simulink model "NLGuidance_12B_with_contracts_SLDV_tmp"  (Simulink 9.0)
settings: Solver=ode3  StartTime=0.0  StopTime=10.0  FixedStep=.02  RelTol=1e-3  EnableMultiTasking=on
model workspace (MAT data in the model file):
  ContractValidatorBlocksMap = containers.Map
  ContractValidatorBlocksMap.serialization.keys = {'NLGuidance_12B/contract/validator', 'NLGuidance_12B_with_contracts/contract/validator'}
  ContractValidatorBlocksMap.serialization.values{1}.block = 'NLGuidance_12B/contract/validator'
  ContractValidatorBlocksMap.serialization.values{1}.assumePorts = 2
  ContractValidatorBlocksMap.serialization.values{1}.guaranteePorts = 6
  ContractValidatorBlocksMap.serialization.values{1}.modeBlocksPorts = 0
  ContractValidatorBlocksMap.serialization.values{1}.portHandles.Inport = [1044.00036621 1045.00036621 1046.00036621 1047.00036621 1048.00036621 1049.00036621 1050.00036621 1051.00036621]
  ContractValidatorBlocksMap.serialization.values{1}.portHandles.Outport = 1052.00036621
  ContractValidatorBlocksMap.serialization.values{1}.portHandles.Enable = []
  ContractValidatorBlocksMap.serialization.values{1}.portHandles.Trigger = []
  ContractValidatorBlocksMap.serialization.values{1}.portHandles.State = []
  ContractValidatorBlocksMap.serialization.values{1}.portHandles.LConn = []
  ContractValidatorBlocksMap.serialization.values{1}.portHandles.RConn = []
  ContractValidatorBlocksMap.serialization.values{1}.portHandles.Ifaction = []
  ContractValidatorBlocksMap.serialization.values{1}.portHandles.Reset = []
  ContractValidatorBlocksMap.serialization.values{1}.portConnectivity(1).Type = '1'
  ContractValidatorBlocksMap.serialization.values{1}.portConnectivity(1).Position = [365 -130]
  ContractValidatorBlocksMap.serialization.values{1}.portConnectivity(1).SrcBlock = 945.000488281
  ContractValidatorBlocksMap.serialization.values{1}.portConnectivity(1).SrcPort = 0
  ContractValidatorBlocksMap.serialization.values{1}.portConnectivity(1).DstBlock = []
  ContractValidatorBlocksMap.serialization.values{1}.portConnectivity(1).DstPort = []
  ContractValidatorBlocksMap.serialization.values{1}.portConnectivity(2).Type = '2'
  ContractValidatorBlocksMap.serialization.values{1}.portConnectivity(2).Position = [365 -40]
  ContractValidatorBlocksMap.serialization.values{1}.portConnectivity(2).SrcBlock = 953.000488281
  ContractValidatorBlocksMap.serialization.values{1}.portConnectivity(2).SrcPort = 0
  ContractValidatorBlocksMap.serialization.values{1}.portConnectivity(2).DstBlock = []
  ContractValidatorBlocksMap.serialization.values{1}.portConnectivity(2).DstPort = []
  ContractValidatorBlocksMap.serialization.values{1}.portConnectivity(3).Type = '3'
  ContractValidatorBlocksMap.serialization.values{1}.portConnectivity(3).Position = [365 50]
  ContractValidatorBlocksMap.serialization.values{1}.portConnectivity(3).SrcBlock = 932.000488281
  ContractValidatorBlocksMap.serialization.values{1}.portConnectivity(3).SrcPort = 0
  ContractValidatorBlocksMap.serialization.values{1}.portConnectivity(3).DstBlock = []
  ContractValidatorBlocksMap.serialization.values{1}.portConnectivity(3).DstPort = []
  ContractValidatorBlocksMap.serialization.values{1}.portConnectivity(4).Type = '4'
  ContractValidatorBlocksMap.serialization.values{1}.portConnectivity(4).Position = [365 140]
  ContractValidatorBlocksMap.serialization.values{1}.portConnectivity(4).SrcBlock = 766.000488281
  ContractValidatorBlocksMap.serialization.values{1}.portConnectivity(4).SrcPort = 0
  ContractValidatorBlocksMap.serialization.values{1}.portConnectivity(4).DstBlock = []
  ContractValidatorBlocksMap.serialization.values{1}.portConnectivity(4).DstPort = []
  ContractValidatorBlocksMap.serialization.values{1}.portConnectivity(5).Type = '5'
  ContractValidatorBlocksMap.serialization.values{1}.portConnectivity(5).Position = [365 230]
  ContractValidatorBlocksMap.serialization.values{1}.portConnectivity(5).SrcBlock = 803.000732422
  ContractValidatorBlocksMap.serialization.values{1}.portConnectivity(5).SrcPort = 0
  ContractValidatorBlocksMap.serialization.values{1}.portConnectivity(5).DstBlock = []
  ContractValidatorBlocksMap.serialization.values{1}.portConnectivity(5).DstPort = []
  ContractValidatorBlocksMap.serialization.values{1}.portConnectivity(6).Type = '6'
  ContractValidatorBlocksMap.serialization.values{1}.portConnectivity(6).Position = [365 320]
  ContractValidatorBlocksMap.serialization.values{1}.portConnectivity(6).SrcBlock = 813.000732422
  ContractValidatorBlocksMap.serialization.values{1}.portConnectivity(6).SrcPort = 0
  ContractValidatorBlocksMap.serialization.values{1}.portConnectivity(6).DstBlock = []
  ContractValidatorBlocksMap.serialization.values{1}.portConnectivity(6).DstPort = []
  ContractValidatorBlocksMap.serialization.values{1}.portConnectivity(7).Type = '7'
  ContractValidatorBlocksMap.serialization.values{1}.portConnectivity(7).Position = [365 410]
  ContractValidatorBlocksMap.serialization.values{1}.portConnectivity(7).SrcBlock = 874.000732422
  ContractValidatorBlocksMap.serialization.values{1}.portConnectivity(7).SrcPort = 0
  ContractValidatorBlocksMap.serialization.values{1}.portConnectivity(7).DstBlock = []
  ContractValidatorBlocksMap.serialization.values{1}.portConnectivity(7).DstPort = []
  ContractValidatorBlocksMap.serialization.values{1}.portConnectivity(8).Type = '8'
  ContractValidatorBlocksMap.serialization.values{1}.portConnectivity(8).Position = [365 500]
  ContractValidatorBlocksMap.serialization.values{1}.portConnectivity(8).SrcBlock = 920.000732422
  ContractValidatorBlocksMap.serialization.values{1}.portConnectivity(8).SrcPort = 0
  ContractValidatorBlocksMap.serialization.values{1}.portConnectivity(8).DstBlock = []
  ContractValidatorBlocksMap.serialization.values{1}.portConnectivity(8).DstPort = []
  ContractValidatorBlocksMap.serialization.values{1}.portConnectivity(9).Type = '1'
  ContractValidatorBlocksMap.serialization.values{1}.portConnectivity(9).Position = [510 185]
  ContractValidatorBlocksMap.serialization.values{1}.portConnectivity(9).SrcBlock = []
  ContractValidatorBlocksMap.serialization.values{1}.portConnectivity(9).SrcPort = []
  ContractValidatorBlocksMap.serialization.values{1}.portConnectivity(9).DstBlock = 962.000488281
  ContractValidatorBlocksMap.serialization.values{1}.portConnectivity(9).DstPort = 0
  ContractValidatorBlocksMap.serialization.values{2}.block = 'NLGuidance_12B_with_contracts/contract/validator'
  ContractValidatorBlocksMap.serialization.values{2}.assumePorts = 2
  ContractValidatorBlocksMap.serialization.values{2}.guaranteePorts = 6
  ContractValidatorBlocksMap.serialization.values{2}.modeBlocksPorts = 0
  ContractValidatorBlocksMap.serialization.values{2}.portHandles.Inport = [4812.00012207 4813.00012207 4814.00012207 4815.00012207 4816.00012207 4817.00012207 4818.00012207 4819.00012207]
  ContractValidatorBlocksMap.serialization.values{2}.portHandles.Outport = 4820.00012207
  ContractValidatorBlocksMap.serialization.values{2}.portHandles.Enable = []
  ContractValidatorBlocksMap.serialization.values{2}.portHandles.Trigger = []
  ContractValidatorBlocksMap.serialization.values{2}.portHandles.State = []
  ContractValidatorBlocksMap.serialization.values{2}.portHandles.LConn = []
  ContractValidatorBlocksMap.serialization.values{2}.portHandles.RConn = []
  ContractValidatorBlocksMap.serialization.values{2}.portHandles.Ifaction = []
  ContractValidatorBlocksMap.serialization.values{2}.portHandles.Reset = []
  ContractValidatorBlocksMap.serialization.values{2}.portConnectivity(1).Type = '1'
  ContractValidatorBlocksMap.serialization.values{2}.portConnectivity(1).Position = [365 -130]
  ContractValidatorBlocksMap.serialization.values{2}.portConnectivity(1).SrcBlock = 4713.00012207
  ContractValidatorBlocksMap.serialization.values{2}.portConnectivity(1).SrcPort = 0
  ContractValidatorBlocksMap.serialization.values{2}.portConnectivity(1).DstBlock = []
  ContractValidatorBlocksMap.serialization.values{2}.portConnectivity(1).DstPort = []
  ContractValidatorBlocksMap.serialization.values{2}.portConnectivity(2).Type = '2'
  ContractValidatorBlocksMap.serialization.values{2}.portConnectivity(2).Position = [365 -40]
  ContractValidatorBlocksMap.serialization.values{2}.portConnectivity(2).SrcBlock = 4721.00012207
  ContractValidatorBlocksMap.serialization.values{2}.portConnectivity(2).SrcPort = 0
  ContractValidatorBlocksMap.serialization.values{2}.portConnectivity(2).DstBlock = []
  ContractValidatorBlocksMap.serialization.values{2}.portConnectivity(2).DstPort = []
  ContractValidatorBlocksMap.serialization.values{2}.portConnectivity(3).Type = '3'
  ContractValidatorBlocksMap.serialization.values{2}.portConnectivity(3).Position = [365 50]
  ContractValidatorBlocksMap.serialization.values{2}.portConnectivity(3).SrcBlock = 4700.00012207
  ContractValidatorBlocksMap.serialization.values{2}.portConnectivity(3).SrcPort = 0
  ContractValidatorBlocksMap.serialization.values{2}.portConnectivity(3).DstBlock = []
  ContractValidatorBlocksMap.serialization.values{2}.portConnectivity(3).DstPort = []
  ContractValidatorBlocksMap.serialization.values{2}.portConnectivity(4).Type = '4'
  ContractValidatorBlocksMap.serialization.values{2}.portConnectivity(4).Position = [365 140]
  ContractValidatorBlocksMap.serialization.values{2}.portConnectivity(4).SrcBlock = 4534.00012207
  ContractValidatorBlocksMap.serialization.values{2}.portConnectivity(4).SrcPort = 0
  ContractValidatorBlocksMap.serialization.values{2}.portConnectivity(4).DstBlock = []
  ContractValidatorBlocksMap.serialization.values{2}.portConnectivity(4).DstPort = []
  ContractValidatorBlocksMap.serialization.values{2}.portConnectivity(5).Type = '5'
  ContractValidatorBlocksMap.serialization.values{2}.portConnectivity(5).Position = [365 230]
  ContractValidatorBlocksMap.serialization.values{2}.portConnectivity(5).SrcBlock = 4571.00012207
  ContractValidatorBlocksMap.serialization.values{2}.portConnectivity(5).SrcPort = 0
  ContractValidatorBlocksMap.serialization.values{2}.portConnectivity(5).DstBlock = []
  ContractValidatorBlocksMap.serialization.values{2}.portConnectivity(5).DstPort = []
  ContractValidatorBlocksMap.serialization.values{2}.portConnectivity(6).Type = '6'
  ContractValidatorBlocksMap.serialization.values{2}.portConnectivity(6).Position = [365 320]
  ContractValidatorBlocksMap.serialization.values{2}.portConnectivity(6).SrcBlock = 4581.00012207
  ContractValidatorBlocksMap.serialization.values{2}.portConnectivity(6).SrcPort = 0
  ContractValidatorBlocksMap.serialization.values{2}.portConnectivity(6).DstBlock = []
  ContractValidatorBlocksMap.serialization.values{2}.portConnectivity(6).DstPort = []
  ContractValidatorBlocksMap.serialization.values{2}.portConnectivity(7).Type = '7'
  ContractValidatorBlocksMap.serialization.values{2}.portConnectivity(7).Position = [365 410]
  ContractValidatorBlocksMap.serialization.values{2}.portConnectivity(7).SrcBlock = 4642.00012207
  ContractValidatorBlocksMap.serialization.values{2}.portConnectivity(7).SrcPort = 0
  ContractValidatorBlocksMap.serialization.values{2}.portConnectivity(7).DstBlock = []
  ContractValidatorBlocksMap.serialization.values{2}.portConnectivity(7).DstPort = []
  ContractValidatorBlocksMap.serialization.values{2}.portConnectivity(8).Type = '8'
  ContractValidatorBlocksMap.serialization.values{2}.portConnectivity(8).Position = [365 500]
  ContractValidatorBlocksMap.serialization.values{2}.portConnectivity(8).SrcBlock = 4688.00012207
  ContractValidatorBlocksMap.serialization.values{2}.portConnectivity(8).SrcPort = 0
  ContractValidatorBlocksMap.serialization.values{2}.portConnectivity(8).DstBlock = []
  ContractValidatorBlocksMap.serialization.values{2}.portConnectivity(8).DstPort = []
  ContractValidatorBlocksMap.serialization.values{2}.portConnectivity(9).Type = '1'
  ContractValidatorBlocksMap.serialization.values{2}.portConnectivity(9).Position = [510 185]
  ContractValidatorBlocksMap.serialization.values{2}.portConnectivity(9).SrcBlock = []
  ContractValidatorBlocksMap.serialization.values{2}.portConnectivity(9).SrcPort = []
  ContractValidatorBlocksMap.serialization.values{2}.portConnectivity(9).DstBlock = 4730.00012207
  ContractValidatorBlocksMap.serialization.values{2}.portConnectivity(9).DstPort = 0
  ContractValidatorBlocksMap.serialization.uniformity = 0
  ContractValidatorBlocksMap.serialization.keyType = 'char'
  ContractValidatorBlocksMap.serialization.valueType = 'any'
libraries: sldvlib x9, simulink x6
settings Model: Creator=elliocm  LastModifiedBy=hbourbou
settings DataIOCC: LimitDataPoints=on  SignalLoggingSaveFormat=ModelDataLogs
settings OptimizationCC: ExpressionDepthLimit=2147483647
settings DebuggingCC: SolverPrmCheckMsg=warning  MultiTaskDSMMsg=warning  MultiTaskCondExecSysMsg=none  StateNameClashWarn=warning
settings GRTTargetCC: GeneratePreprocessorConditionals=Disable all
settings ConfigComp: DVMode=PropertyProving  DVMaxProcessTime=7200  DVTestSuiteOptimization=CombinedObjectives (Nonlinear Extended)

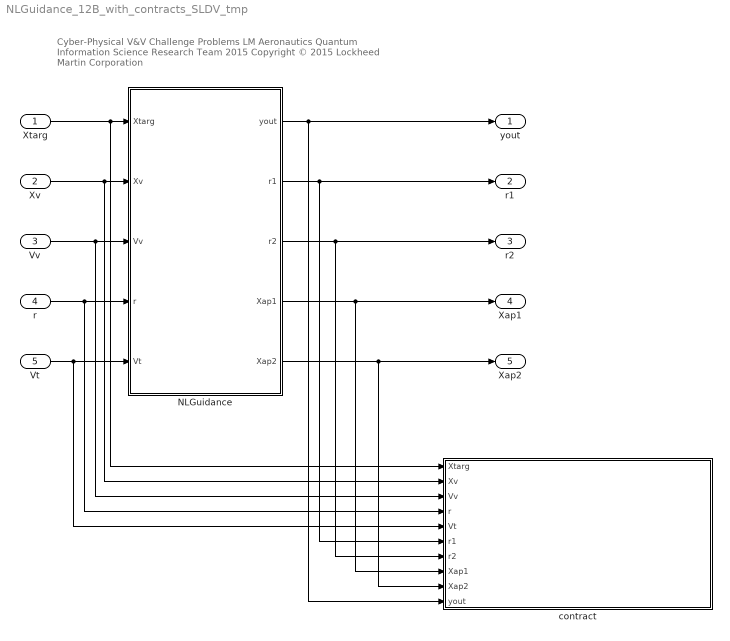
== system NLGuidance_12B_with_contracts_SLDV_tmp ==
  note: Cyber-Physical V&V Challenge Problems
      | LM Aeronautics Quantum Information Science Research Team 2015
      | Copyright © 2015 Lockheed Martin Corporation
  Xtarg : Inport  OutDataTypeStr=double  PortDimensions=3
  Xv : Inport  Port=2  OutDataTypeStr=double  PortDimensions=3
  Vv : Inport  Port=3  OutDataTypeStr=double  PortDimensions=3
  r : Inport  Port=4  OutDataTypeStr=double
  Vt : Inport  Port=5  OutDataTypeStr=double  PortDimensions=3
  NLGuidance : Subsystem
  contract : Subsystem  TreatAsAtomicUnit=on  mask(VerificationSubsystem){}
      settings: CopyFcn=set_param(gcb, 'LinkStatus', 'none');
      mask Display: image(imread('sldvicon_versubsys.png','BackGroundColor',[1 1 1]),'center');
  yout : Outport  VectorParamsAs1DForOutWhenUnconnected=off
  r1 : Outport  Port=2  VectorParamsAs1DForOutWhenUnconnected=off
  r2 : Outport  Port=3  VectorParamsAs1DForOutWhenUnconnected=off
  Xap1 : Outport  Port=4  VectorParamsAs1DForOutWhenUnconnected=off
  Xap2 : Outport  Port=5  VectorParamsAs1DForOutWhenUnconnected=off
  wires:
  NLGuidance/1(yout) -> contract/10(yout), yout/1
  Xv/1 -> contract/2(Xv), NLGuidance/2(Xv)
  Vv/1 -> contract/3(Vv), NLGuidance/3(Vv)
  r/1 -> contract/4(r), NLGuidance/4(r)
  Vt/1 -> contract/5(Vt), NLGuidance/5(Vt)
  Xtarg/1 -> contract/1(Xtarg), NLGuidance/1(Xtarg)
  NLGuidance/3(r2) -> contract/7(r2), r2/1
  NLGuidance/4(Xap1) -> contract/8(Xap1), Xap1/1
  NLGuidance/5(Xap2) -> contract/9(Xap2), Xap2/1
  NLGuidance/2(r1) -> contract/6(r1), r1/1

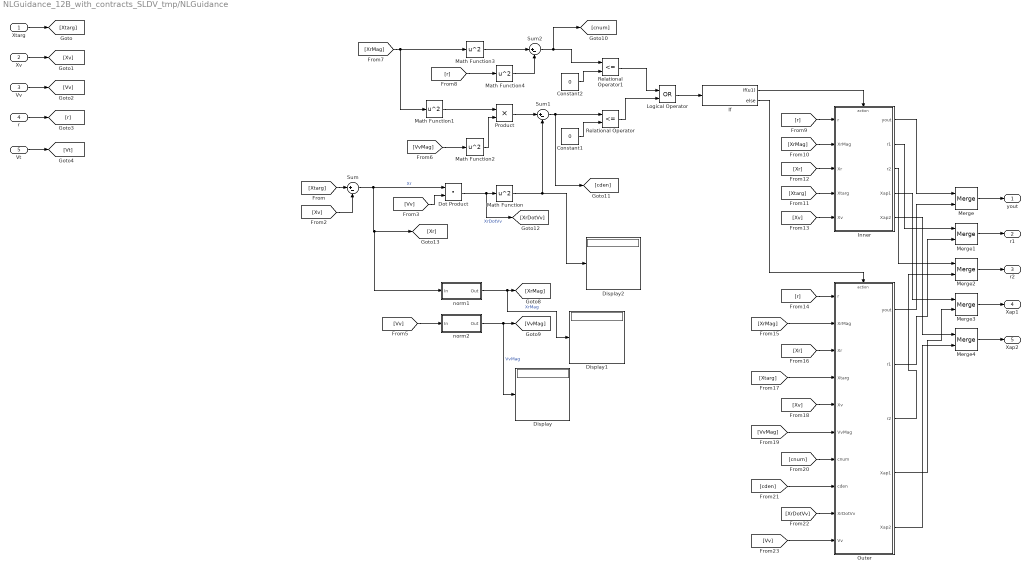
== system NLGuidance_12B_with_contracts_SLDV_tmp/NLGuidance ==
  Xtarg : Inport
  Xv : Inport  Port=2
  Vv : Inport  Port=3
  r : Inport  Port=4
  Vt : Inport  Port=5
  Constant1 : Constant  Value=0
  Constant2 : Constant  Value=0
  Display : Display
  Display1 : Display
  Display2 : Display
  Dot Product : DotProduct  InputSameDT=on  OutDataTypeStr=Inherit: Inherit via internal rule
  If : If  IfExpression=u1
  Inner : Subsystem
  Logical Operator : Logic  Operator=OR  AllPortsSameDT=off  OutDataTypeStr=boolean
  Math Function{,1..4} (5 alike) : Math  Operator=square  SaturateOnIntegerOverflow=on
  Merge{,1..4} (5 alike) : Merge
  Outer : Subsystem
  Product : Product  RndMeth=Zero
  Relational Operator : RelationalOperator  Operator=<=  OutDataTypeStr=boolean  RndMeth=Nearest
  Relational Operator1 : RelationalOperator  Operator=<=  OutDataTypeStr=boolean  RndMeth=Nearest
  Sum : Sum  Inputs=|+-
  Sum1 : Sum  Inputs=|+-
  Sum2 : Sum  Inputs=|+-
  norm1 : Subsystem
  norm2 : Subsystem
  yout : Outport  VectorParamsAs1DForOutWhenUnconnected=off
  r1 : Outport  Port=2  VectorParamsAs1DForOutWhenUnconnected=off
  r2 : Outport  Port=3  VectorParamsAs1DForOutWhenUnconnected=off
  Xap1 : Outport  Port=4  VectorParamsAs1DForOutWhenUnconnected=off
  Xap2 : Outport  Port=5  VectorParamsAs1DForOutWhenUnconnected=off
  wires:
  Xtarg/1 -> [Xtarg]
  Xv/1 -> [Xv]
  Vv/1 -> [Vv]
  r/1 -> [r]
  Vt/1 -> [Vt]
  [Xtarg] -> Sum/1
  [Xv] -> Sum/2
  Sum/1 -> norm1/1(In), [Xr], Dot Product/1  "Xr"
  [Vv] -> Dot Product/2
  Dot Product/1 -> [XrDotVv], Math Function/1  "XrDotVv"
  norm1/1(Out) -> Display1/1, [XrMag]  "XrMag"
  [Vv] -> norm2/1(In)
  norm2/1(Out) -> Display/1, [VvMag]  "VvMag"
  Math Function/1 -> Display2/1, Sum1/2
  [VvMag] -> Math Function2/1
  Math Function1/1 -> Product/1
  Math Function2/1 -> Product/2
  Product/1 -> Sum1/1
  Sum1/1 -> [cden], Relational Operator/1
  Constant1/1 -> Relational Operator/2
  Relational Operator/1 -> Logical Operator/2
  Sum2/1 -> [cnum], Relational Operator1/1
  Constant2/1 -> Relational Operator1/2
  Relational Operator1/1 -> Logical Operator/1
  Math Function3/1 -> Sum2/1
  [XrMag] -> Math Function1/1, Math Function3/1
  Math Function4/1 -> Sum2/2
  [r] -> Math Function4/1
  [r] -> Inner/1(r)
  [XrMag] -> Inner/2(XrMag)
  Logical Operator/1 -> If/1
  [Xtarg] -> Inner/4(Xtarg)
  [Xr] -> Inner/3(Xr)
  [Xv] -> Inner/5(Xv)
  Inner/1(yout) -> Merge/1
  Outer/1(yout) -> Merge/2
  If/1 -> Inner/Action
  If/2 -> Outer/Action
  [r] -> Outer/1(r)
  [XrMag] -> Outer/2(XrMag)
  [Xr] -> Outer/3(Xr)
  [Xtarg] -> Outer/4(Xtarg)
  [Xv] -> Outer/5(Xv)
  [VvMag] -> Outer/6(VvMag)
  [cnum] -> Outer/7(cnum)
  [cden] -> Outer/8(cden)
  [XrDotVv] -> Outer/9(XrDotVv)
  [Vv] -> Outer/10(Vv)
  Merge/1 -> yout/1
  Merge1/1 -> r1/1
  Inner/2(r1) -> Merge1/1
  Outer/2(r1) -> Merge1/2
  Merge2/1 -> r2/1
  Outer/3(r2) -> Merge2/2
  Inner/3(r2) -> Merge2/1
  Merge3/1 -> Xap1/1
  Merge4/1 -> Xap2/1
  Inner/4(Xap1) -> Merge3/1
  Outer/4(Xap1) -> Merge3/2
  Inner/5(Xap2) -> Merge4/1
  Outer/5(Xap2) -> Merge4/2

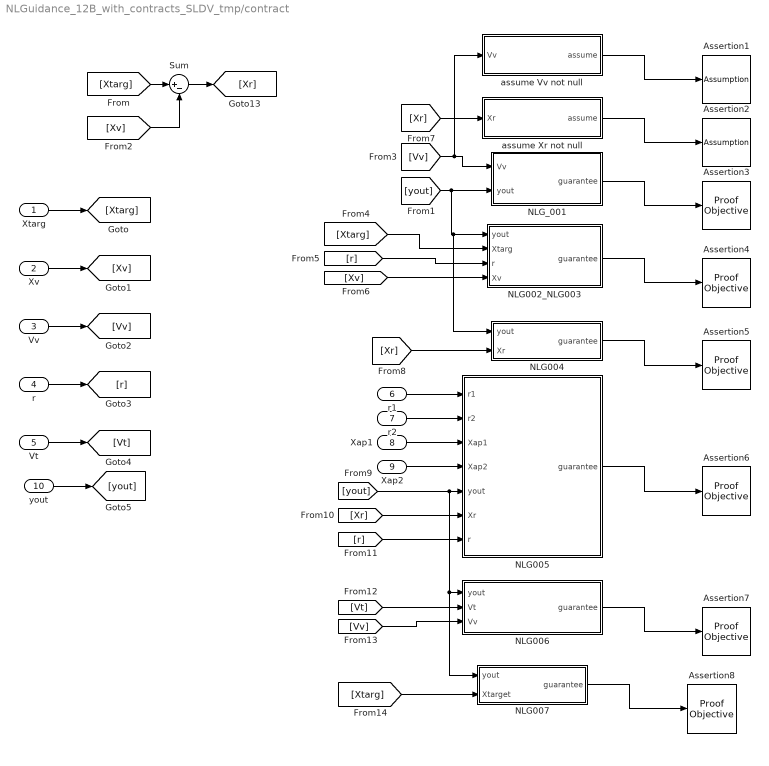
== system NLGuidance_12B_with_contracts_SLDV_tmp/contract ==
  Xtarg : Inport  OutDataTypeStr=double  PortDimensions=3
  Xv : Inport  Port=2  OutDataTypeStr=double  PortDimensions=3
  Vv : Inport  Port=3  OutDataTypeStr=double  PortDimensions=3
  r : Inport  Port=4  OutDataTypeStr=double
  Vt : Inport  Port=5  OutDataTypeStr=double  PortDimensions=3
  r1 : Inport  Port=6
  r2 : Inport  Port=7
  Xap1 : Inport  Port=8
  Xap2 : Inport  Port=9
  yout : Inport  Port=10
  Assertion1 : sldvlib/Objectives and Constraints/Assumption  enabled=on  customAVTBlockType=Assumption  intervals=true  initial=off  dispValues=on  outEnabled=off
      settings: AttributesFormatString=%<intervals>  SourceProductName=Simulink  SourceProductBaseCode=SL
  Assertion2 : sldvlib/Objectives and Constraints/Assumption  enabled=on  customAVTBlockType=Assumption  intervals=true  initial=off  dispValues=on  outEnabled=off
      settings: AttributesFormatString=%<intervals>  SourceProductName=Simulink  SourceProductBaseCode=SL
  Assertion{3..8} (6 alike) : sldvlib/Objectives and Constraints/Proof Objective  enabled=on  customAVTBlockType=Proof Objective  intervals=true  dispValues=on  outEnabled=off  enableStopSim=off
      settings: AttributesFormatString=%<intervals>  SourceProductName=Simulink  SourceProductBaseCode=SL
  NLG002_NLG003 : Subsystem
  NLG004 : Subsystem
  NLG005 : Subsystem
  NLG006 : Subsystem
  NLG007 : Subsystem
  NLG_001 : Subsystem
  Sum : Sum  Inputs=|+-
  assume Vv not null : Subsystem
  assume Xr not null : Subsystem
  wires:
  Xtarg/1 -> [Xtarg]
  Xv/1 -> [Xv]
  Vv/1 -> [Vv]
  Vt/1 -> [Vt]
  r/1 -> [r]
  [Xv] -> Sum/2
  [Xtarg] -> Sum/1
  Sum/1 -> [Xr]
  [yout] -> NLG004/1(yout), NLG002_NLG003/1(yout), NLG_001/2(yout)
  [Vv] -> assume Vv not null/1(Vv), NLG_001/1(Vv)
  yout/1 -> [yout]
  [Xtarg] -> NLG002_NLG003/2(Xtarg)
  [r] -> NLG002_NLG003/3(r)
  [Xv] -> NLG002_NLG003/4(Xv)
  [Xr] -> assume Xr not null/1(Xr)
  [Xr] -> NLG004/2(Xr)
  r1/1 -> NLG005/1(r1)
  r2/1 -> NLG005/2(r2)
  Xap1/1 -> NLG005/3(Xap1)
  Xap2/1 -> NLG005/4(Xap2)
  [yout] -> NLG007/1(yout), NLG006/1(yout), NLG005/5(yout)
  [Xr] -> NLG005/6(Xr)
  [r] -> NLG005/7(r)
  [Vt] -> NLG006/2(Vt)
  [Vv] -> NLG006/3(Vv)
  [Xtarg] -> NLG007/2(Xtarget)
  assume Vv not null/1(assume) -> Assertion1/1
  assume Xr not null/1(assume) -> Assertion2/1
  NLG_001/1(guarantee) -> Assertion3/1
  NLG002_NLG003/1(guarantee) -> Assertion4/1
  NLG004/1(guarantee) -> Assertion5/1
  NLG005/1(guarantee) -> Assertion6/1
  NLG006/1(guarantee) -> Assertion7/1
  NLG007/1(guarantee) -> Assertion8/1

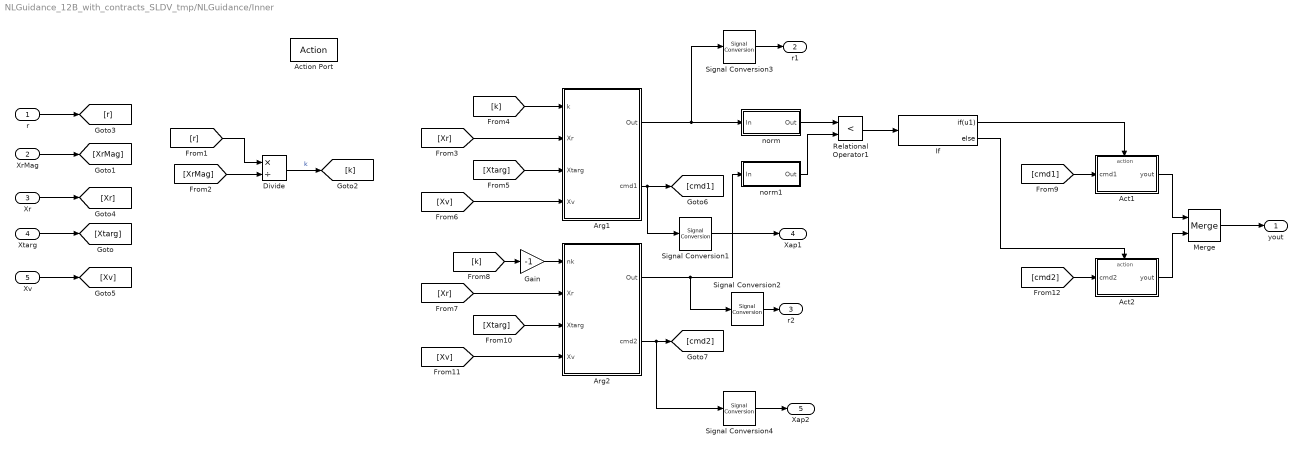
== system NLGuidance_12B_with_contracts_SLDV_tmp/NLGuidance/Inner ==
  r : Inport
  XrMag : Inport  Port=2
  Xr : Inport  Port=3
  Xtarg : Inport  Port=4
  Xv : Inport  Port=5
  Action Port : ActionPort
  Act1 : Subsystem
  Act2 : Subsystem
  Arg1 : Subsystem
  Arg2 : Subsystem
  Divide : Product  Inputs=*/
  Gain : Gain  Gain=-1
  If : If  IfExpression=u1
  Merge : Merge
  Relational Operator1 : RelationalOperator  Operator=<  OutDataTypeStr=boolean  RndMeth=Nearest
  Signal Conversion{1..4} (4 alike) : SignalConversion  OverrideOpt=off
  norm : Subsystem
  norm1 : Subsystem
  yout : Outport  VectorParamsAs1DForOutWhenUnconnected=off
  r1 : Outport  Port=2  VectorParamsAs1DForOutWhenUnconnected=off
  r2 : Outport  Port=3  VectorParamsAs1DForOutWhenUnconnected=off
  Xap1 : Outport  Port=4  VectorParamsAs1DForOutWhenUnconnected=off
  Xap2 : Outport  Port=5  VectorParamsAs1DForOutWhenUnconnected=off
  wires:
  Divide/1 -> [k]  "k"
  r/1 -> [r]
  XrMag/1 -> [XrMag]
  Xtarg/1 -> [Xtarg]
  [r] -> Divide/1
  [XrMag] -> Divide/2
  Xr/1 -> [Xr]
  Xv/1 -> [Xv]
  norm/1(Out) -> Relational Operator1/1
  norm1/1(Out) -> Relational Operator1/2
  Arg1/1(Out) -> Signal Conversion3/1, norm/1(In)
  [k] -> Arg1/1(k)
  [Xr] -> Arg1/2(Xr)
  [Xtarg] -> Arg1/3(Xtarg)
  [Xv] -> Arg1/4(Xv)
  Relational Operator1/1 -> If/1
  [Xr] -> Arg2/2(Xr)
  [Xtarg] -> Arg2/3(Xtarg)
  [Xv] -> Arg2/4(Xv)
  Arg2/1(Out) -> Signal Conversion2/1, norm1/1(In)
  [k] -> Gain/1
  Gain/1 -> Arg2/1(nk)
  Arg1/2(cmd1) -> Signal Conversion1/1, [cmd1]
  [cmd1] -> Act1/1(cmd1)
  [cmd2] -> Act2/1(cmd2)
  Act1/1(yout) -> Merge/1
  Act2/1(yout) -> Merge/2
  Merge/1 -> yout/1
  If/1 -> Act1/Action
  If/2 -> Act2/Action
  Arg2/2(cmd2) -> Signal Conversion4/1, [cmd2]
  Signal Conversion3/1 -> r1/1
  Signal Conversion1/1 -> Xap1/1
  Signal Conversion2/1 -> r2/1
  Signal Conversion4/1 -> Xap2/1

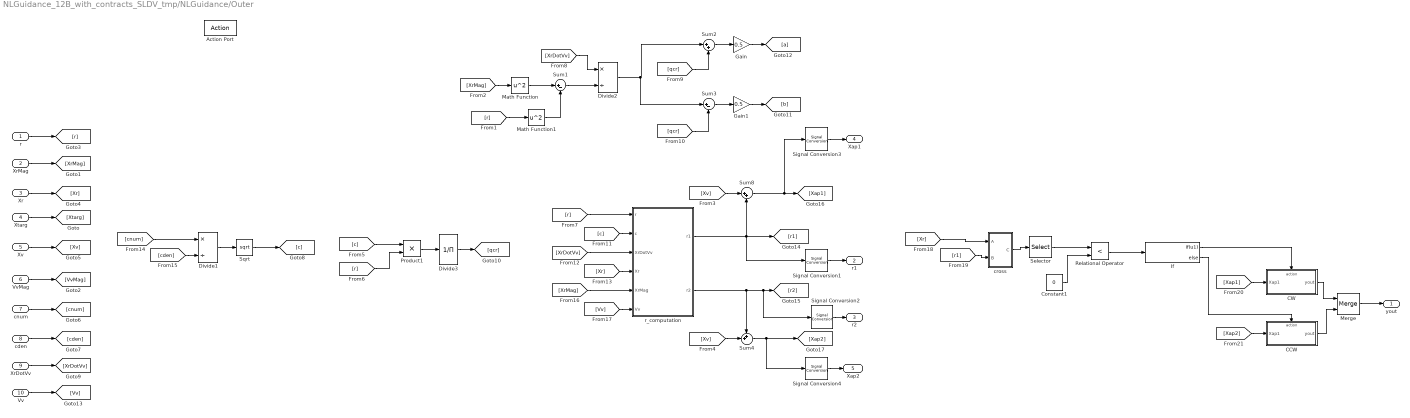
== system NLGuidance_12B_with_contracts_SLDV_tmp/NLGuidance/Outer ==
  r : Inport
  XrMag : Inport  Port=2
  Xr : Inport  Port=3
  Xtarg : Inport  Port=4
  Xv : Inport  Port=5
  VvMag : Inport  Port=6
  cnum : Inport  Port=7
  cden : Inport  Port=8
  XrDotVv : Inport  Port=9
  Vv : Inport  Port=10
  Action Port : ActionPort
  CCW : Subsystem
  CW : Subsystem
  Constant1 : Constant  Value=0
  Divide1 : Product  Inputs=*/
  Divide2 : Product  Inputs=*/
  Divide3 : Product  Inputs=/
  Gain : Gain  Gain=0.5
  Gain1 : Gain  Gain=0.5
  If : If  IfExpression=u1
  Math Function : Math  Operator=square  SaturateOnIntegerOverflow=on
  Math Function1 : Math  Operator=square  SaturateOnIntegerOverflow=on
  Merge : Merge
  Product1 : Product
  Relational Operator : RelationalOperator  Operator=<  OutDataTypeStr=boolean  RndMeth=Nearest
  Selector : Selector  InputPortWidth=3  IndexOptions=Index vector (dialog)  Indices=[3]  OutputSizes=1
  Signal Conversion{1..4} (4 alike) : SignalConversion  OverrideOpt=off
  Sqrt : Sqrt  SaturateOnIntegerOverflow=on
  Sum1 : Sum  Inputs=|+-
  Sum2 : Sum  Inputs=|++
  Sum3 : Sum  Inputs=|+-
  Sum4 : Sum  Inputs=++|
  Sum8 : Sum  Inputs=|++
  cross : Subsystem
  r_computation : Subsystem
  yout : Outport  VectorParamsAs1DForOutWhenUnconnected=off
  r1 : Outport  Port=2  VectorParamsAs1DForOutWhenUnconnected=off
  r2 : Outport  Port=3  VectorParamsAs1DForOutWhenUnconnected=off
  Xap1 : Outport  Port=4  VectorParamsAs1DForOutWhenUnconnected=off
  Xap2 : Outport  Port=5  VectorParamsAs1DForOutWhenUnconnected=off
  wires:
  r/1 -> [r]
  XrMag/1 -> [XrMag]
  Xtarg/1 -> [Xtarg]
  Xr/1 -> [Xr]
  Xv/1 -> [Xv]
  [XrMag] -> Math Function/1
  [r] -> Math Function1/1
  VvMag/1 -> [VvMag]
  cnum/1 -> [cnum]
  [cnum] -> Divide1/1
  [cden] -> Divide1/2
  Divide1/1 -> Sqrt/1
  Sqrt/1 -> [c]
  cden/1 -> [cden]
  XrDotVv/1 -> [XrDotVv]
  [c] -> Product1/1
  [r] -> Product1/2
  Math Function/1 -> Sum1/1
  Math Function1/1 -> Sum1/2
  Sum1/1 -> Divide2/2
  [XrDotVv] -> Divide2/1
  Divide2/1 -> Sum3/1, Sum2/1
  Sum2/1 -> Gain/1
  Sum3/1 -> Gain1/1
  Product1/1 -> Divide3/1
  Divide3/1 -> [qcr]
  [qcr] -> Sum2/2
  [qcr] -> Sum3/2
  Gain1/1 -> [b]
  Gain/1 -> [a]
  Vv/1 -> [Vv]
  r_computation/1(r1) -> Signal Conversion1/1, Sum8/2, [r1]
  r_computation/2(r2) -> Sum4/1, Signal Conversion2/1, [r2]
  [Xv] -> Sum8/1
  [Xv] -> Sum4/2
  Sum8/1 -> Signal Conversion3/1, [Xap1]
  Sum4/1 -> Signal Conversion4/1, [Xap2]
  [r] -> r_computation/1(r)
  [c] -> r_computation/2(c)
  [XrDotVv] -> r_computation/3(XrDotVv)
  [Xr] -> r_computation/4(Xr)
  [XrMag] -> r_computation/5(XrMag)
  [Vv] -> r_computation/6(Vv)
  cross/1(C) -> Selector/1
  [Xr] -> cross/1(A)
  [r1] -> cross/2(B)
  Constant1/1 -> Relational Operator/2
  Selector/1 -> Relational Operator/1
  Relational Operator/1 -> If/1
  If/1 -> CW/Action
  [Xap1] -> CW/1(Xap1)
  If/2 -> CCW/Action
  [Xap2] -> CCW/1(Xap1)
  CW/1(yout) -> Merge/1
  CCW/1(yout) -> Merge/2
  Merge/1 -> yout/1
  Signal Conversion3/1 -> Xap1/1
  Signal Conversion1/1 -> r1/1
  Signal Conversion2/1 -> r2/1
  Signal Conversion4/1 -> Xap2/1

== system NLGuidance_12B_with_contracts_SLDV_tmp/NLGuidance/norm1 ==
  In : Inport
  Math Function : Math  Operator=square  SaturateOnIntegerOverflow=on
  Math Function1 : Math  Operator=sqrt  SaturateOnIntegerOverflow=on
  Sum of Elements : Sum  Inputs=+
  Out : Outport  VectorParamsAs1DForOutWhenUnconnected=off
  wires:
  Math Function/1 -> Sum of Elements/1
  Sum of Elements/1 -> Math Function1/1
  In/1 -> Math Function/1
  Math Function1/1 -> Out/1

== system NLGuidance_12B_with_contracts_SLDV_tmp/NLGuidance/norm2 ==
  In : Inport
  Math Function : Math  Operator=square  SaturateOnIntegerOverflow=on
  Math Function1 : Math  Operator=sqrt  SaturateOnIntegerOverflow=on
  Sum of Elements : Sum  Inputs=+
  Out : Outport  VectorParamsAs1DForOutWhenUnconnected=off
  wires:
  Math Function1/1 -> Out/1
  In/1 -> Math Function/1
  Sum of Elements/1 -> Math Function1/1
  Math Function/1 -> Sum of Elements/1

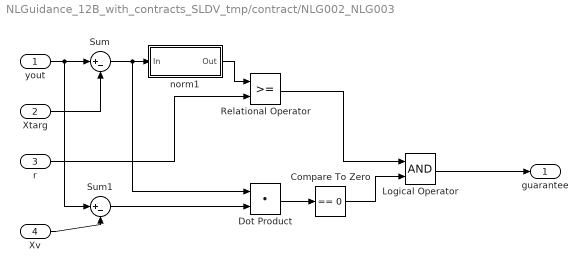
== system NLGuidance_12B_with_contracts_SLDV_tmp/contract/NLG002_NLG003 ==
  yout : Inport
  Xtarg : Inport  Port=2
  r : Inport  Port=3
  Xv : Inport  Port=4
  Compare To Zero : simulink/Logic and Bit Operations/Compare To Zero  relop===  OutDataTypeStr=boolean
  Dot Product : DotProduct  InputSameDT=on  OutDataTypeStr=Inherit: Inherit via internal rule
  Logical Operator : Logic  AllPortsSameDT=off  OutDataTypeStr=boolean
  Relational Operator : RelationalOperator  OutDataTypeStr=boolean  RndMeth=Simplest
  Sum : Sum  Inputs=|+-
  Sum1 : Sum  Inputs=|+-
  norm1 : Subsystem
  guarantee : Outport  OutDataTypeStr=boolean  VectorParamsAs1DForOutWhenUnconnected=off
  wires:
  Logical Operator/1 -> guarantee/1
  Xtarg/1 -> Sum/2
  yout/1 -> Sum1/1, Sum/1
  Sum/1 -> Dot Product/1, norm1/1(In)
  norm1/1(Out) -> Relational Operator/1
  r/1 -> Relational Operator/2
  Relational Operator/1 -> Logical Operator/1
  Xv/1 -> Sum1/2
  Sum1/1 -> Dot Product/2
  Dot Product/1 -> Compare To Zero/1
  Compare To Zero/1 -> Logical Operator/2

== system NLGuidance_12B_with_contracts_SLDV_tmp/contract/NLG004 ==
  yout : Inport
  Xr : Inport  Port=2
  Compare To Zero : simulink/Logic and Bit Operations/Compare To Zero  relop=>  OutDataTypeStr=boolean
  Dot Product : DotProduct  InputSameDT=on  OutDataTypeStr=Inherit: Inherit via internal rule
  guarantee : Outport  OutDataTypeStr=boolean  VectorParamsAs1DForOutWhenUnconnected=off
  wires:
  Compare To Zero/1 -> guarantee/1
  Dot Product/1 -> Compare To Zero/1
  yout/1 -> Dot Product/1
  Xr/1 -> Dot Product/2

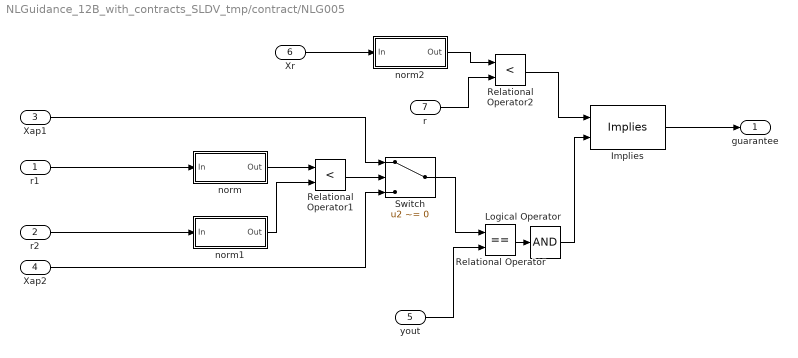
== system NLGuidance_12B_with_contracts_SLDV_tmp/contract/NLG005 ==
  r1 : Inport
  r2 : Inport  Port=2
  Xap1 : Inport  Port=3
  Xap2 : Inport  Port=4
  yout : Inport  Port=5
  Xr : Inport  Port=6
  r : Inport  Port=7
  Implies : sldvlib/Verification Utilities/Implies
      settings: SourceProductName=Simulink Design Verifier  SourceProductBaseCode=DV
  Logical Operator : Logic  Inputs=1  AllPortsSameDT=off  OutDataTypeStr=boolean
  Relational Operator : RelationalOperator  Operator===  OutDataTypeStr=boolean  RndMeth=Simplest
  Relational Operator1 : RelationalOperator  Operator=<  OutDataTypeStr=boolean  RndMeth=Nearest
  Relational Operator2 : RelationalOperator  Operator=<  OutDataTypeStr=boolean  RndMeth=Nearest
  Switch : Switch  Criteria=u2 ~= 0
  norm : Subsystem
  norm1 : Subsystem
  norm2 : Subsystem
  guarantee : Outport  OutDataTypeStr=boolean  VectorParamsAs1DForOutWhenUnconnected=off
  wires:
  norm/1(Out) -> Relational Operator1/1
  norm1/1(Out) -> Relational Operator1/2
  r1/1 -> norm/1(In)
  r2/1 -> norm1/1(In)
  Relational Operator1/1 -> Switch/2
  Xap1/1 -> Switch/1
  Xap2/1 -> Switch/3
  Switch/1 -> Relational Operator/1
  yout/1 -> Relational Operator/2
  Relational Operator/1 -> Logical Operator/1
  Logical Operator/1 -> Implies/2
  Implies/1 -> guarantee/1
  Xr/1 -> norm2/1(In)
  norm2/1(Out) -> Relational Operator2/1
  r/1 -> Relational Operator2/2
  Relational Operator2/1 -> Implies/1

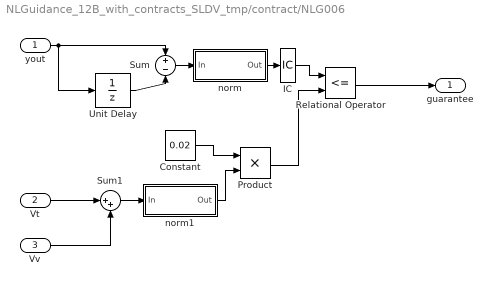
== system NLGuidance_12B_with_contracts_SLDV_tmp/contract/NLG006 ==
  yout : Inport
  Vt : Inport  Port=2
  Vv : Inport  Port=3
  Constant : Constant  Value=0.02  SampleTime=-1
  IC : InitialCondition  Value=0
  Product : Product
  Relational Operator : RelationalOperator  Operator=<=  OutDataTypeStr=boolean  RndMeth=Simplest
  Sum : Sum  Inputs=+-
  Sum1 : Sum  Inputs=|++
  Unit Delay : UnitDelay  SampleTime=-1  HasFrameUpgradeWarning=on
  norm : Subsystem
  norm1 : Subsystem
  guarantee : Outport  OutDataTypeStr=boolean  VectorParamsAs1DForOutWhenUnconnected=off
  wires:
  yout/1 -> Unit Delay/1, Sum/1
  Unit Delay/1 -> Sum/2
  Sum/1 -> norm/1(In)
  norm/1(Out) -> IC/1
  Constant/1 -> Product/1
  norm1/1(Out) -> Product/2
  Sum1/1 -> norm1/1(In)
  Vt/1 -> Sum1/1
  Vv/1 -> Sum1/2
  Product/1 -> Relational Operator/2
  Relational Operator/1 -> guarantee/1
  IC/1 -> Relational Operator/1

== system NLGuidance_12B_with_contracts_SLDV_tmp/contract/NLG007 ==
  yout : Inport
  Xtarget : Inport  Port=2
  Compare To Zero : simulink/Logic and Bit Operations/Compare To Zero  relop===  OutDataTypeStr=boolean
  Selector : Selector  InputPortWidth=3  IndexOptions=Index vector (dialog)  Indices=3  OutputSizes=1
  Sum : Sum  Inputs=|+-
  guarantee : Outport  OutDataTypeStr=boolean  VectorParamsAs1DForOutWhenUnconnected=off
  wires:
  Compare To Zero/1 -> guarantee/1
  Sum/1 -> Selector/1
  yout/1 -> Sum/1
  Xtarget/1 -> Sum/2
  Selector/1 -> Compare To Zero/1

== system NLGuidance_12B_with_contracts_SLDV_tmp/contract/NLG_001 ==
  Vv : Inport
  yout : Inport  Port=2
  Compare To Zero : simulink/Logic and Bit Operations/Compare To Zero  relop=>  OutDataTypeStr=boolean
  Product : Product
  Sum : Sum  Inputs=1
  guarantee : Outport  OutDataTypeStr=boolean  VectorParamsAs1DForOutWhenUnconnected=off
  wires:
  Vv/1 -> Product/1
  yout/1 -> Product/2
  Product/1 -> Sum/1
  Sum/1 -> Compare To Zero/1
  Compare To Zero/1 -> guarantee/1

== system NLGuidance_12B_with_contracts_SLDV_tmp/contract/assume Vv not null ==
  Vv : Inport
  Compare To Zero : simulink/Logic and Bit Operations/Compare To Zero  relop=~=  OutDataTypeStr=boolean
  all : Logic  Inputs=1  AllPortsSameDT=off  OutDataTypeStr=boolean
  assume : Outport  OutDataTypeStr=boolean  VectorParamsAs1DForOutWhenUnconnected=off
  wires:
  all/1 -> assume/1
  Vv/1 -> Compare To Zero/1
  Compare To Zero/1 -> all/1

== system NLGuidance_12B_with_contracts_SLDV_tmp/contract/assume Xr not null ==
  Xr : Inport
  Compare To Zero : simulink/Logic and Bit Operations/Compare To Zero  relop=~=  OutDataTypeStr=boolean
  all : Logic  Inputs=1  AllPortsSameDT=off  OutDataTypeStr=boolean
  assume : Outport  OutDataTypeStr=boolean  VectorParamsAs1DForOutWhenUnconnected=off
  wires:
  Xr/1 -> Compare To Zero/1
  Compare To Zero/1 -> all/1
  all/1 -> assume/1

== system NLGuidance_12B_with_contracts_SLDV_tmp/NLGuidance/Inner/Act1 ==
  cmd1 : Inport
  Action Port : ActionPort
  yout : Outport  VectorParamsAs1DForOutWhenUnconnected=off
  wires:
  cmd1/1 -> yout/1

== system NLGuidance_12B_with_contracts_SLDV_tmp/NLGuidance/Inner/Act2 ==
  cmd2 : Inport
  Action Port : ActionPort
  yout : Outport  VectorParamsAs1DForOutWhenUnconnected=off
  wires:
  cmd2/1 -> yout/1

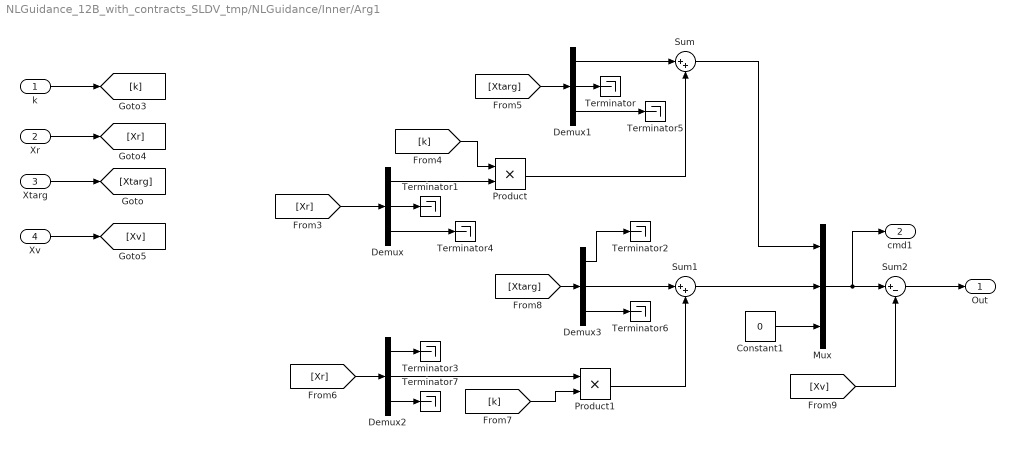
== system NLGuidance_12B_with_contracts_SLDV_tmp/NLGuidance/Inner/Arg1 ==
  k : Inport
  Xr : Inport  Port=2
  Xtarg : Inport  Port=3
  Xv : Inport  Port=4
  Constant1 : Constant  Value=0
  Demux{,1..3} (4 alike) : Demux  Outputs=3
  Mux : Mux  Inputs=3
  Product : Product  RndMeth=Zero
  Product1 : Product  RndMeth=Zero
  Sum : Sum  Inputs=|++
  Sum1 : Sum  Inputs=|++
  Sum2 : Sum  Inputs=|+-
  Terminator{,1..7} (8 alike) : Terminator
  Out : Outport  VectorParamsAs1DForOutWhenUnconnected=off
  cmd1 : Outport  Port=2  VectorParamsAs1DForOutWhenUnconnected=off
  wires:
  Mux/1 -> cmd1/1, Sum2/1
  Demux3/3 -> Terminator6/1
  Demux/2 -> Terminator1/1
  [Xr] -> Demux2/1
  Sum/1 -> Mux/1
  Demux1/2 -> Terminator/1
  [k] -> Product1/2
  Constant1/1 -> Mux/3
  Demux3/2 -> Sum1/1
  Demux2/1 -> Terminator3/1
  [Xtarg] -> Demux1/1
  Product/1 -> Sum/2
  [k] -> Product/1
  Demux/1 -> Product/2
  [Xr] -> Demux/1
  Sum1/1 -> Mux/2
  Demux1/1 -> Sum/1
  Demux2/3 -> Terminator7/1
  [Xtarg] -> Demux3/1
  Sum2/1 -> Out/1
  Demux/3 -> Terminator4/1
  [Xv] -> Sum2/2
  Demux3/1 -> Terminator2/1
  Demux2/2 -> Product1/1
  Product1/1 -> Sum1/2
  Demux1/3 -> Terminator5/1
  k/1 -> [k]
  Xtarg/1 -> [Xtarg]
  Xr/1 -> [Xr]
  Xv/1 -> [Xv]

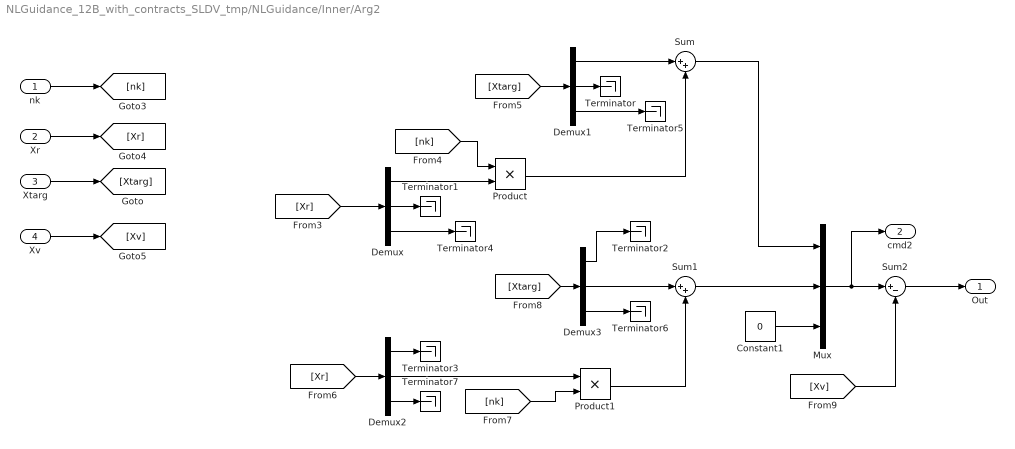
== system NLGuidance_12B_with_contracts_SLDV_tmp/NLGuidance/Inner/Arg2 ==
  nk : Inport
  Xr : Inport  Port=2
  Xtarg : Inport  Port=3
  Xv : Inport  Port=4
  Constant1 : Constant  Value=0
  Demux{,1..3} (4 alike) : Demux  Outputs=3
  Mux : Mux  Inputs=3
  Product : Product  RndMeth=Zero
  Product1 : Product  RndMeth=Zero
  Sum : Sum  Inputs=|++
  Sum1 : Sum  Inputs=|++
  Sum2 : Sum  Inputs=|+-
  Terminator{,1..7} (8 alike) : Terminator
  Out : Outport  VectorParamsAs1DForOutWhenUnconnected=off
  cmd2 : Outport  Port=2  VectorParamsAs1DForOutWhenUnconnected=off
  wires:
  Xv/1 -> [Xv]
  Xr/1 -> [Xr]
  Xtarg/1 -> [Xtarg]
  nk/1 -> [nk]
  Demux1/3 -> Terminator5/1
  Product1/1 -> Sum1/2
  Demux2/2 -> Product1/1
  Demux3/1 -> Terminator2/1
  [Xv] -> Sum2/2
  Demux/3 -> Terminator4/1
  Sum2/1 -> Out/1
  [Xtarg] -> Demux3/1
  Demux2/3 -> Terminator7/1
  Demux1/1 -> Sum/1
  Sum1/1 -> Mux/2
  [Xr] -> Demux/1
  Demux/1 -> Product/2
  [nk] -> Product/1
  Product/1 -> Sum/2
  [Xtarg] -> Demux1/1
  Demux2/1 -> Terminator3/1
  Demux3/2 -> Sum1/1
  Constant1/1 -> Mux/3
  [nk] -> Product1/2
  Demux1/2 -> Terminator/1
  Sum/1 -> Mux/1
  [Xr] -> Demux2/1
  Demux/2 -> Terminator1/1
  Demux3/3 -> Terminator6/1
  Mux/1 -> cmd2/1, Sum2/1

== system NLGuidance_12B_with_contracts_SLDV_tmp/NLGuidance/Inner/norm ==
  In : Inport
  Math Function : Math  Operator=square  SaturateOnIntegerOverflow=on
  Math Function1 : Math  Operator=sqrt  SaturateOnIntegerOverflow=on
  Sum of Elements : Sum  Inputs=+
  Out : Outport  VectorParamsAs1DForOutWhenUnconnected=off
  wires:
  Math Function1/1 -> Out/1
  In/1 -> Math Function/1
  Sum of Elements/1 -> Math Function1/1
  Math Function/1 -> Sum of Elements/1

== system NLGuidance_12B_with_contracts_SLDV_tmp/NLGuidance/Inner/norm1 ==
  In : Inport
  Math Function : Math  Operator=square  SaturateOnIntegerOverflow=on
  Math Function1 : Math  Operator=sqrt  SaturateOnIntegerOverflow=on
  Sum of Elements : Sum  Inputs=+
  Out : Outport  VectorParamsAs1DForOutWhenUnconnected=off
  wires:
  Math Function/1 -> Sum of Elements/1
  Sum of Elements/1 -> Math Function1/1
  In/1 -> Math Function/1
  Math Function1/1 -> Out/1

== system NLGuidance_12B_with_contracts_SLDV_tmp/NLGuidance/Outer/CCW ==
  Xap1 : Inport
  Action Port : ActionPort
  yout : Outport  VectorParamsAs1DForOutWhenUnconnected=off
  wires:
  Xap1/1 -> yout/1

== system NLGuidance_12B_with_contracts_SLDV_tmp/NLGuidance/Outer/CW ==
  Xap1 : Inport
  Action Port : ActionPort
  yout : Outport  VectorParamsAs1DForOutWhenUnconnected=off
  wires:
  Xap1/1 -> yout/1

== system NLGuidance_12B_with_contracts_SLDV_tmp/NLGuidance/Outer/cross ==
  A : Inport
  B : Inport  Port=2
  A_1 : InportShadow
  B_1 : InportShadow  Port=2
  Subsystem1 : Subsystem
  Subsystem2 : Subsystem
  Sum : Sum  Inputs=+|-  SaturateOnIntegerOverflow=on  InputSameDT=on  OutDataTypeStr=Inherit: Same as first input
  C : Outport  VectorParamsAs1DForOutWhenUnconnected=off
  wires:
  B/1 -> Subsystem2/2(B1)
  A_1/1 -> Subsystem1/1(A1)
  A/1 -> Subsystem2/1(A1)
  Subsystem2/1(Out1) -> Sum/1
  B_1/1 -> Subsystem1/2(B1)
  Sum/1 -> C/1
  Subsystem1/1(Out1) -> Sum/2

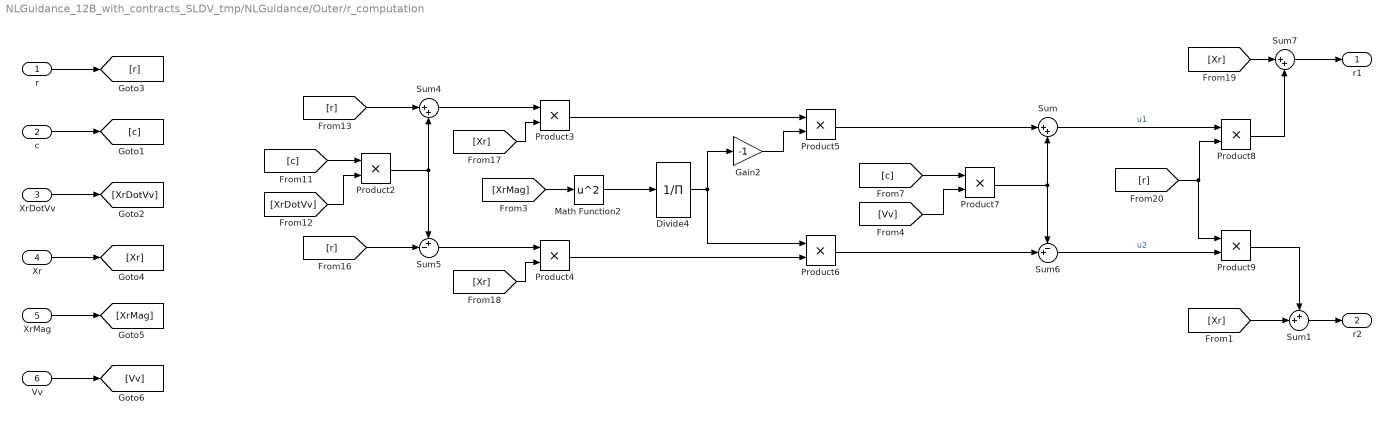
== system NLGuidance_12B_with_contracts_SLDV_tmp/NLGuidance/Outer/r_computation ==
  r : Inport
  c : Inport  Port=2
  XrDotVv : Inport  Port=3
  Xr : Inport  Port=4
  XrMag : Inport  Port=5
  Vv : Inport  Port=6
  Divide4 : Product  Inputs=/
  Gain2 : Gain  Gain=-1
  Math Function2 : Math  Operator=square  SaturateOnIntegerOverflow=on
  Product{2..9} (8 alike) : Product
  Sum : Sum  Inputs=|++
  Sum1 : Sum  Inputs=++|
  Sum4 : Sum  Inputs=|++
  Sum5 : Sum  Inputs=+-|
  Sum6 : Sum  Inputs=-+|
  Sum7 : Sum  Inputs=|++
  r1 : Outport  VectorParamsAs1DForOutWhenUnconnected=off
  r2 : Outport  Port=2  VectorParamsAs1DForOutWhenUnconnected=off
  wires:
  [r] -> Sum4/1
  Sum6/1 -> Product9/2  "u2"
  Gain2/1 -> Product5/2
  Product4/1 -> Product6/2
  [XrDotVv] -> Product2/2
  [Xr] -> Product4/2
  Product3/1 -> Product5/1
  Divide4/1 -> Product6/1, Gain2/1
  Sum5/1 -> Product4/1
  [Xr] -> Sum7/1
  [Vv] -> Product7/2
  Product7/1 -> Sum/2, Sum6/1
  [r] -> Product9/1, Product8/2
  Product8/1 -> Sum7/2
  Sum7/1 -> r1/1
  Product6/1 -> Sum6/2
  Product5/1 -> Sum/1
  [Xr] -> Product3/2
  [c] -> Product7/1
  Math Function2/1 -> Divide4/1
  [XrMag] -> Math Function2/1
  [c] -> Product2/1
  Sum4/1 -> Product3/1
  Sum/1 -> Product8/1  "u1"
  Product2/1 -> Sum5/1, Sum4/2
  [r] -> Sum5/2
  r/1 -> [r]
  c/1 -> [c]
  XrDotVv/1 -> [XrDotVv]
  Xr/1 -> [Xr]
  XrMag/1 -> [XrMag]
  Vv/1 -> [Vv]
  Product9/1 -> Sum1/1
  [Xr] -> Sum1/2
  Sum1/1 -> r2/1

== system NLGuidance_12B_with_contracts_SLDV_tmp/contract/NLG002_NLG003/norm1 ==
  In : Inport
  Math Function : Math  Operator=square  SaturateOnIntegerOverflow=on
  Math Function1 : Math  Operator=sqrt  SaturateOnIntegerOverflow=on
  Sum of Elements : Sum  Inputs=+
  Out : Outport  VectorParamsAs1DForOutWhenUnconnected=off
  wires:
  Math Function/1 -> Sum of Elements/1
  Sum of Elements/1 -> Math Function1/1
  In/1 -> Math Function/1
  Math Function1/1 -> Out/1

== system NLGuidance_12B_with_contracts_SLDV_tmp/contract/NLG005/norm ==
  In : Inport
  Math Function : Math  Operator=square  SaturateOnIntegerOverflow=on
  Math Function1 : Math  Operator=sqrt  SaturateOnIntegerOverflow=on
  Sum of Elements : Sum  Inputs=+
  Out : Outport  VectorParamsAs1DForOutWhenUnconnected=off
  wires:
  Math Function1/1 -> Out/1
  In/1 -> Math Function/1
  Sum of Elements/1 -> Math Function1/1
  Math Function/1 -> Sum of Elements/1

== system NLGuidance_12B_with_contracts_SLDV_tmp/contract/NLG005/norm1 ==
  In : Inport
  Math Function : Math  Operator=square  SaturateOnIntegerOverflow=on
  Math Function1 : Math  Operator=sqrt  SaturateOnIntegerOverflow=on
  Sum of Elements : Sum  Inputs=+
  Out : Outport  VectorParamsAs1DForOutWhenUnconnected=off
  wires:
  Math Function/1 -> Sum of Elements/1
  Sum of Elements/1 -> Math Function1/1
  In/1 -> Math Function/1
  Math Function1/1 -> Out/1

== system NLGuidance_12B_with_contracts_SLDV_tmp/contract/NLG005/norm2 ==
  In : Inport
  Math Function : Math  Operator=square  SaturateOnIntegerOverflow=on
  Math Function1 : Math  Operator=sqrt  SaturateOnIntegerOverflow=on
  Sum of Elements : Sum  Inputs=+
  Out : Outport  VectorParamsAs1DForOutWhenUnconnected=off
  wires:
  Math Function1/1 -> Out/1
  In/1 -> Math Function/1
  Sum of Elements/1 -> Math Function1/1
  Math Function/1 -> Sum of Elements/1

== system NLGuidance_12B_with_contracts_SLDV_tmp/contract/NLG006/norm ==
  In : Inport
  Math Function : Math  Operator=square  SaturateOnIntegerOverflow=on
  Math Function1 : Math  Operator=sqrt  SaturateOnIntegerOverflow=on
  Sum of Elements : Sum  Inputs=+
  Out : Outport  VectorParamsAs1DForOutWhenUnconnected=off
  wires:
  Math Function1/1 -> Out/1
  In/1 -> Math Function/1
  Sum of Elements/1 -> Math Function1/1
  Math Function/1 -> Sum of Elements/1

== system NLGuidance_12B_with_contracts_SLDV_tmp/contract/NLG006/norm1 ==
  In : Inport
  Math Function : Math  Operator=square  SaturateOnIntegerOverflow=on
  Math Function1 : Math  Operator=sqrt  SaturateOnIntegerOverflow=on
  Sum of Elements : Sum  Inputs=+
  Out : Outport  VectorParamsAs1DForOutWhenUnconnected=off
  wires:
  Math Function1/1 -> Out/1
  In/1 -> Math Function/1
  Sum of Elements/1 -> Math Function1/1
  Math Function/1 -> Sum of Elements/1

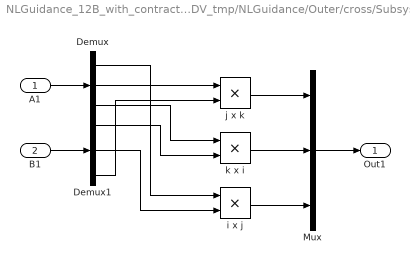
== system NLGuidance_12B_with_contracts_SLDV_tmp/NLGuidance/Outer/cross/Subsystem1 ==
  A1 : Inport
  B1 : Inport  Port=2
  Demux : Demux  Outputs=3
  Demux1 : Demux  Outputs=3
  Mux : Mux  Inputs=3
  i x j : Product  SaturateOnIntegerOverflow=on  InputSameDT=on  OutDataTypeStr=Inherit: Same as first input
  j x k : Product  SaturateOnIntegerOverflow=on  InputSameDT=on  OutDataTypeStr=Inherit: Same as first input
  k x i : Product  SaturateOnIntegerOverflow=on  InputSameDT=on  OutDataTypeStr=Inherit: Same as first input
  Out1 : Outport  VectorParamsAs1DForOutWhenUnconnected=off
  wires:
  Demux/2 -> j x k/1
  Demux1/3 -> j x k/2
  A1/1 -> Demux/1
  Demux/3 -> k x i/1
  Mux/1 -> Out1/1
  j x k/1 -> Mux/1
  B1/1 -> Demux1/1
  k x i/1 -> Mux/2
  Demux1/2 -> i x j/2
  i x j/1 -> Mux/3
  Demux/1 -> i x j/1
  Demux1/1 -> k x i/2

== system NLGuidance_12B_with_contracts_SLDV_tmp/NLGuidance/Outer/cross/Subsystem2 ==
  A1 : Inport
  B1 : Inport  Port=2
  Demux : Demux  Outputs=3
  Demux1 : Demux  Outputs=3
  Mux : Mux  Inputs=3
  i x j : Product  SaturateOnIntegerOverflow=on  InputSameDT=on  OutDataTypeStr=Inherit: Same as first input
  j x k : Product  SaturateOnIntegerOverflow=on  InputSameDT=on  OutDataTypeStr=Inherit: Same as first input
  k x i : Product  SaturateOnIntegerOverflow=on  InputSameDT=on  OutDataTypeStr=Inherit: Same as first input
  Out1 : Outport  VectorParamsAs1DForOutWhenUnconnected=off
  wires:
  Demux1/1 -> k x i/2
  Demux/1 -> i x j/1
  i x j/1 -> Mux/3
  Demux1/2 -> i x j/2
  k x i/1 -> Mux/2
  B1/1 -> Demux1/1
  j x k/1 -> Mux/1
  Mux/1 -> Out1/1
  Demux/3 -> k x i/1
  A1/1 -> Demux/1
  Demux1/3 -> j x k/2
  Demux/2 -> j x k/1
